simulink model "probl4_lab1"  (Simulink 6.0)
settings: Solver=ode45  StartTime=0.0  StopTime=100.0  RelTol=1e-3
undefined symbols (not defined in the file): kr, Ti
settings Model: LastModifiedBy=student

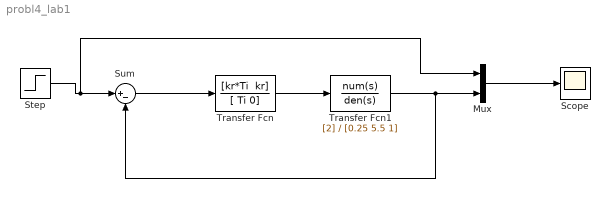
== system probl4_lab1 ==
  Mux : Mux  Inputs=2
  Scope : Scope
  Step : Step  SampleTime=0
  Sum : Sum  Inputs=|+-
  Transfer Fcn : TransferFcn  Numerator="[kr*Ti  kr]"  Denominator=[ Ti 0]
  Transfer Fcn1 : TransferFcn  Numerator=[2]  Denominator=[0.25 5.5 1]
  wires:
  Step/1 -> Sum/1, Mux/1
  Sum/1 -> Transfer Fcn/1
  Transfer Fcn/1 -> Transfer Fcn1/1
  Mux/1 -> Scope/1
  Transfer Fcn1/1 -> Mux/2, Sum/2
